simulink model "performMission"  (R2016a)
settings: Solver=VariableStepAuto  StartTime=0.0  StopTime=400  FixedStep=0.001  RelTol=1e-3
InitFcn:
  | workspaceVariablesPerformMission
values from neighbouring files (symbols this model uses):
  ac_id = 127    [goToMission_enu.m]    (also in messageListener.m = 126; workspaceVariablesPerformMissionBackup.m = 202)
  destinations1 = [depot(1,:) ... (first row only)    [workspaceVariablesPerformMission.m]    (also in workspaceVariablesPerformMissionBackup.m = [depot1)
  destinations2 = [depot(2,:) ... (first row only)    [workspaceVariablesPerformMission.m]    (also in workspaceVariablesPerformMissionBackup.m = [depot2)
  pprz_id = 153    [workspaceVariablesPerformMissionBackup.m]
  Q = 3    [workspaceVariablesPerformMission.m]    (also in workspaceVariablesPerformMissionBackup.m)
  wp_ids = [4 5 6 7]    [workspaceVariablesPerformMission.m]    (also in workspaceVariablesPerformMissionBackup.m)
libraries: dspnetwork x4, realtime_pacer_lib x2
settings Model: Creator=pulkit  LastModifiedBy=Kuldeep

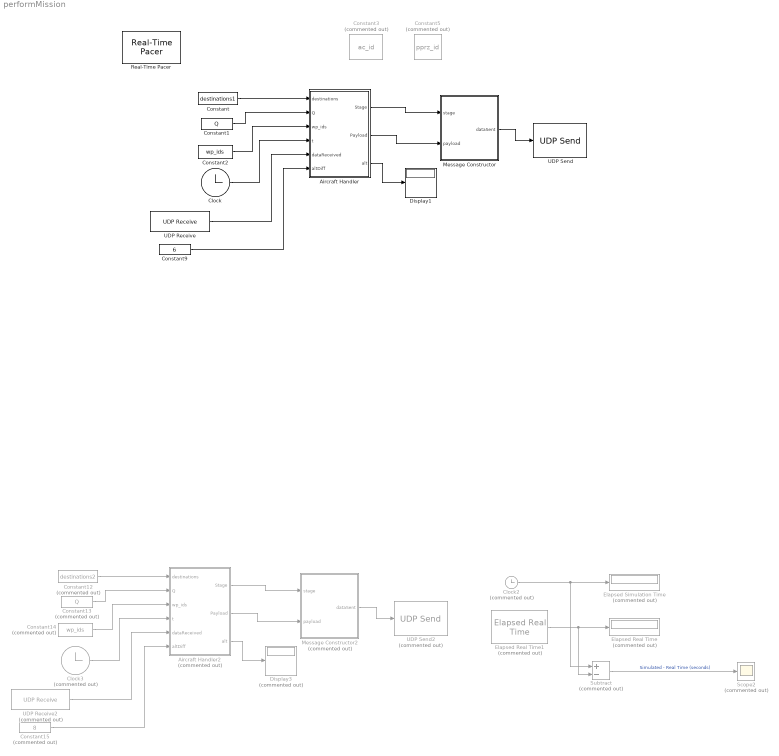
== system performMission ==
  Aircraft Handler : MATLAB Function  TreatAsAtomicUnit=on
  Aircraft Handler2 : MATLAB Function  Commented=on  TreatAsAtomicUnit=on
  Clock : Clock
  Clock2 : Clock  Commented=on
  Clock3 : Clock  Commented=on
  Constant : Constant  Value=destinations1  VectorParams1D=off
  Constant1 : Constant  Value=Q  VectorParams1D=off
  Constant12 : Constant  Commented=on  Value=destinations2  VectorParams1D=off
  Constant13 : Constant  Commented=on  Value=Q  VectorParams1D=off
  Constant14 : Constant  Commented=on  Value=wp_ids  VectorParams1D=off
  Constant15 : Constant  Commented=on  Value=8  VectorParams1D=off
  Constant2 : Constant  Value=wp_ids  VectorParams1D=off
  Constant3 : Constant  Commented=on  Value=ac_id  VectorParams1D=off
  Constant5 : Constant  Commented=on  Value=pprz_id  VectorParams1D=off
  Constant9 : Constant  Value=6  VectorParams1D=off
  Display1 : Display
  Display3 : Display  Commented=on
  Elapsed Real Time : Display  Commented=on
      settings: Decimation=2
  Elapsed Real Time1 : realtime_pacer_lib/Elapsed Real Time  Commented=on
  Elapsed Simulation Time : Display  Commented=on
      settings: Decimation=2
  Message Constructor : MATLAB Function  TreatAsAtomicUnit=on
  Message Constructor2 : MATLAB Function  Commented=on  TreatAsAtomicUnit=on
  Real-Time Pacer : realtime_pacer_lib/Real-Time Pacer  simTimePerRealTime=1
  Scope2 : Scope  Commented=on
  Subtract : Sum  Commented=on  Inputs=+-
  UDP Receive : dspnetwork/UDP Receive  localURL='0.0.0.0'  localPort=4142  remoteURL='0.0.0.0'  remotePort=-1  recvBufferSize=8192  dims=255  signalDatatype=uint8  isVarSize=on  showBlockingTime=on  blockingTime=0.  sampletime=0.005  blockPlatform=HOST
  UDP Receive2 : dspnetwork/UDP Receive  Commented=on  localURL='0.0.0.0'  localPort=4042  remoteURL='0.0.0.0'  remotePort=-1  recvBufferSize=8192  dims=255  signalDatatype=uint8  isVarSize=on  showBlockingTime=on  blockingTime=0.  sampletime=0.005  blockPlatform=HOST
  UDP Send : dspnetwork/UDP Send  remoteURL='255.255.255.255'  remotePort=4143  localURL='0.0.0.0'  localPortSource=Automatically determine  localPort=-1  sampletime=-1  blockPlatform=HOST  separateLengthPort=0
  UDP Send2 : dspnetwork/UDP Send  Commented=on  remoteURL='255.255.255.255'  remotePort=4043  localURL='0.0.0.0'  localPortSource=Automatically determine  localPort=-1  sampletime=-1  blockPlatform=HOST  separateLengthPort=0
  wires:
  Clock/1 -> Aircraft Handler/4(t)
  Constant/1 -> Aircraft Handler/1(destinations)
  Constant1/1 -> Aircraft Handler/2(Q)
  Constant2/1 -> Aircraft Handler/3(wp_ids)
  Aircraft Handler/1(Stage) -> Message Constructor/1(stage)
  Aircraft Handler/2(Payload) -> Message Constructor/2(payload)
  Message Constructor/1(dataSent) -> UDP Send/1
  UDP Receive/1 -> Aircraft Handler/5(dataReceived)
  Clock2/1 -> Subtract/1, Elapsed Simulation Time/1
  Subtract/1 -> Scope2/1  "Simulated - Real Time (seconds)"
  Elapsed Real Time1/1 -> Subtract/2, Elapsed Real Time/1
  Constant9/1 -> Aircraft Handler/6(altDiff)
  Aircraft Handler/3(alt) -> Display1/1
  ? -> ?
  Clock3/1 -> Aircraft Handler2/4(t)
  Constant12/1 -> Aircraft Handler2/1(destinations)
  Constant13/1 -> Aircraft Handler2/2(Q)
  Constant14/1 -> Aircraft Handler2/3(wp_ids)
  Aircraft Handler2/1(Stage) -> Message Constructor2/1(stage)
  Aircraft Handler2/2(Payload) -> Message Constructor2/2(payload)
  Message Constructor2/1(dataSent) -> UDP Send2/1
  UDP Receive2/1 -> Aircraft Handler2/5(dataReceived)
  Constant15/1 -> Aircraft Handler2/6(altDiff)
  Aircraft Handler2/3(alt) -> Display3/1

== matlab function performMission/Aircraft Handler ==
  settings: updateMethod=DISCRETE  sampleTime=0.001
  data: Stage output size=1; destinations input; Payload output size=[1 5]; Q input; wp_ids input; t input; dataReceived input uint8; altDiff input size=[1 1]; alt output size=[1 1]
function [Stage, Payload, alt] = fcn(destinations, Q, wp_ids, t, dataReceived, altDiff)
%#codegen
% This file determines what stage the vehicle is in and forwards the
% appropriate payload. If payload is empty, then no data is sent.

% Following stages are possible:
% % Stage 0 - Initialization (e.g. reading INS_REF)
% % Stage 1 - Event of WP movement i.e. send "MOVE_WP" as payload
% % Stage 2 - Event of instructing vehicle to start following the route i.e.
% send "BLOCK" as payload
% % Stage 3 - Listening when to start the next route. This is decided by
% the user in the flight plan

%% Persistent variables definition
persistent ct_route tStep ct_WP isRouteFinished tol stage stateChange presentRoute alt0 payloadSent

%% Initialize the persistent variables
% % ct_customer - customer number in route for which the WP is being moved

% % ct_route idefies which route number is being currently traversed by the
% vehicle

if isempty(ct_WP)
    ct_WP = 1;
end
if isempty(tStep)
    tStep = 5;
end
if isempty(isRouteFinished)
    isRouteFinished = 1;
end
if isempty(tol)
    tol = 0.001;
end
if isempty(stage)
    stage = 0;
end
if isempty(presentRoute)
    presentRoute = 1;
end
if isempty(ct_route)
    ct_route = 1;
end
if isempty(alt0)
    alt0 = 0;
end
if isempty(payloadSent)
    payloadSent = 0;
end

stateChange = 0;
alt = alt0+altDiff;
ac_id = 126;
block_id = 3; % Start engine block in the flight plan
%% 
% if isRouteFinished && ~isempty(dataReceived) && dataReceived(4)==24
%     val = typecast(dataReceived(5:8), 'single');
%     if abs(val)<tol
%         isRouteFinished = 0;
%     end
% end

% ct_route = floor(t/tStep)+1;

if ct_route <= (size(destinations,1)-1)/Q
    route = [destinations(1,:); destinations((ct_route-1)*Q+2:ct_route*Q+1,:)];
else
    route = destinations(1:Q+1,:);
end

Payload = zeros(1,0);
if stage == 0
    % % Reading the value of reference altitude corresponding to the ground
    % from INS_REF telemetry message
    if ~isempty(dataReceived) && dataReceived(3)==ac_id && dataReceived(4)==154
        alt0 = double(typecast(dataReceived(29:32), 'int32')/1000); % Reading hmsl0
        stage = 40;
        stateChange = 1;
    end
    
elseif stage == 10 % % Update WP for the depot and customers in a route
    % % Move next WP only if the movement of the previous one is confirmed
    % TO DO - change payloadSent to 0 after few seconds (in case message 47
    % is not picked up by the listener)
%     if ~payloadSent
%         coordinates = [route(ct_WP,1:2) alt];
%         wp_id = wp_ids(ct_WP);
%         Payload = [wp_id, ac_id, coordinates];
%         payloadSent = 1;
        
    if ~isempty(dataReceived) && dataReceived(3)==ac_id && dataReceived(4)==47 && dataReceived(5)==wp_ids(ct_WP)
        val = typecast(dataReceived(6:9), 'int32'); % lat
        val1 = typecast(dataReceived(10:13), 'int32'); % lon
        if abs(val-route(ct_WP,1)*10^7)<100 && abs(val1-route(ct_WP,2)*10^7) <100
        %     ct_customer = rem(ct_customer,Q)+1;
            ct_WP = ct_WP + 1;
            if ct_WP > Q+1
                ct_WP = 1;
                stage = 30; 
                stateChange = 1;
            end
        end
        payloadSent = 0;
    end
    coordinates = [route(ct_WP,1:2) alt];
    wp_id = wp_ids(ct_WP);
    Payload = [wp_id, ac_id, coordinates];
    
    
elseif stage == 20 % % Wait for the confirmation from the user to initiate route
    
    
elseif stage == 30 % % Send Start-Engine message and confirm that it happened
    if ~isempty(dataReceived) && dataReceived(3)==ac_id && dataReceived(4)==217
        val = typecast(dataReceived(5:8), 'single');
        if abs(val)<tol % If drone has initiated its route
            stage = 40;
            stateChange = 1;
        else % Send start-engine message
            Payload = [block_id, ac_id];
        end
    end
        
elseif stage == 40 % % Listening till user confirms that drone is ready for next-route
    if ~isempty(dataReceived) && dataReceived(3)==ac_id && dataReceived(4)==217
        val = typecast(dataReceived(5:8), 'single');
        if abs(val-1)<tol
            stage = 10;
            stateChange = 1;
            
            % To change to next route
            ct_route = ct_route+1;
        end
    end
    
end

Stage = stage;
% In case of change in state, the payload is reset to be empty to avoid any
% discrepencies in the datalink message
if stateChange
    Payload = zeros(1,0);
end

== matlab function performMission/Message Constructor ==
  settings: updateMethod=DISCRETE  sampleTime=0.001
  data: stage input; payload input; dataSent output uint8 size=[1 20]
function dataSent = fcn(stage, payload)
%#codegen
% pprz_id - The Paparazzi message ID (Default 153 - Don't change)
% message_id - Message ID of the data to be sent through downlink
% dataL_payload - Length of the payload in Number of bytes (uint8) required
% ac_id - ID of the aircraft to which the message is to be sent
% payload - The actual data to be sent via datalink
% stage - The stage (defined in previous function) at which the present UAV is in
% 
dataSent = uint8(zeros(1,0));
if ~isempty(payload)
    pprz_id = 153;
    dataL_overhead = 4 + 2; % Number of bytes (unint8) required as overhead on actual data
    if stage == 10
        % Construct MOVE_WP message
        message_id = 2;
        dataL_payload = 2 + 4*3;
        dataSent = [uint8(pprz_id) uint8(dataL_overhead+dataL_payload) uint8(0) uint8(message_id) ...
                uint8(payload(1:2)) typecast(int32(payload(3)*10^7),'uint8') typecast(int32(payload(4)*10^7),'uint8') typecast(int32(payload(5)*10^3),'uint8')];
    elseif stage == 30
        % Contruct BLOCK message
        message_id = 5;
        dataL_payload = 2;
        dataSent = [uint8(pprz_id) uint8(dataL_overhead+dataL_payload) uint8(0) uint8(message_id) ...
            uint8(payload(1:2))];
    end

    % Add CHECKSUM if its a useful datalink message
    ck_a = uint8(0);
    ck_b = uint8(0);
    for i=2:dataSent(2)-2
        ck_a = uint8(rem(uint16(ck_a)+uint16(dataSent(i)),uint16(256)));
        ck_b = uint8(rem(uint16(ck_b)+uint16(ck_a),uint16(256)));
    end
    dataSent = typecast([dataSent ck_a ck_b],'uint8');
else
    dataSent = uint8(zeros(1,0));
end

== matlab function performMission/Aircraft Handler2 ==
  settings: updateMethod=DISCRETE  sampleTime=0.001
  data: Stage output size=1; destinations input; Payload output size=[1 5]; Q input; wp_ids input; t input; dataReceived input uint8; altDiff input size=[1 1]; alt output size=[1 1]
function [Stage, Payload, alt] = fcn(destinations, Q, wp_ids, t, dataReceived, altDiff)
%#codegen
% This file determines what stage the vehicle is in and forwards the
% appropriate payload. If payload is empty, then no data is sent.

% Following stages are possible:
% % Stage 0 - Initialization (e.g. reading INS_REF)
% % Stage 1 - Event of WP movement i.e. send "MOVE_WP" as payload
% % Stage 2 - Event of instructing vehicle to start following the route i.e.
% send "BLOCK" as payload
% % Stage 3 - Listening when to start the next route. This is decided by
% the user in the flight plan

%% Persistent variables definition
persistent ct_route tStep ct_WP isRouteFinished tol stage stateChange presentRoute alt0 payloadSent

%% Initialize the persistent variables
% % ct_customer - customer number in route for which the WP is being moved

% % ct_route idefies which route number is being currently traversed by the
% vehicle

if isempty(ct_WP)
    ct_WP = 1;
end
if isempty(tStep)
    tStep = 5;
end
if isempty(isRouteFinished)
    isRouteFinished = 1;
end
if isempty(tol)
    tol = 0.001;
end
if isempty(stage)
    stage = 0;
end
if isempty(presentRoute)
    presentRoute = 1;
end
if isempty(ct_route)
    ct_route = 1;
end
if isempty(alt0)
    alt0 = 0;
end
if isempty(payloadSent)
    payloadSent = 0;
end

stateChange = 0;
alt = alt0+altDiff;
ac_id = 127;
block_id = 3; % Start engine block in the flight plan
%% 
% if isRouteFinished && ~isempty(dataReceived) && dataReceived(4)==24
%     val = typecast(dataReceived(5:8), 'single');
%     if abs(val)<tol
%         isRouteFinished = 0;
%     end
% end

% ct_route = floor(t/tStep)+1;

if ct_route <= (size(destinations,1)-1)/Q
    route = [destinations(1,:); destinations((ct_route-1)*Q+2:ct_route*Q+1,:)];
else
    route = destinations(1:Q+1,:);
end

Payload = zeros(1,0);
if stage == 0
    % % Reading the value of reference altitude corresponding to the ground
    % from INS_REF telemetry message
    if ~isempty(dataReceived) && dataReceived(3)==ac_id && dataReceived(4)==154
        alt0 = double(typecast(dataReceived(29:32), 'int32')/1000); % Reading hmsl0
        stage = 40;
        stateChange = 1;
    end
    
elseif stage == 10 % % Update WP for the depot and customers in a route
    % % Move next WP only if the movement of the previous one is confirmed
    % TO DO - change payloadSent to 0 after few seconds (in case message 47
    % is not picked up by the listener)
%     if ~payloadSent
%         coordinates = [route(ct_WP,1:2) alt];
%         wp_id = wp_ids(ct_WP);
%         Payload = [wp_id, ac_id, coordinates];
%         payloadSent = 1;
        
    if ~isempty(dataReceived) && dataReceived(3)==ac_id && dataReceived(4)==47 && dataReceived(5)==wp_ids(ct_WP)
        val = typecast(dataReceived(6:9), 'int32'); % lat
        val1 = typecast(dataReceived(10:13), 'int32'); % lon
        if abs(val-route(ct_WP,1)*10^7)<100 && abs(val1-route(ct_WP,2)*10^7) <100
        %     ct_customer = rem(ct_customer,Q)+1;
            ct_WP = ct_WP + 1;
            if ct_WP > Q+1
                ct_WP = 1;
                stage = 30; 
                stateChange = 1;
            end
        end
        payloadSent = 0;
    end
    coordinates = [route(ct_WP,1:2) alt];
    wp_id = wp_ids(ct_WP);
    Payload = [wp_id, ac_id, coordinates];
    
    
elseif stage == 20 % % Wait for the confirmation from the user to initiate route
    
    
elseif stage == 30 % % Send Start-Engine message and confirm that it happened
    if ~isempty(dataReceived) && dataReceived(3)==ac_id && dataReceived(4)==217
        val = typecast(dataReceived(5:8), 'single');
        if abs(val)<tol % If drone has initiated its route
            stage = 40;
            stateChange = 1;
        else % Send start-engine message
            Payload = [block_id, ac_id];
        end
    end
        
elseif stage == 40 % % Listening till user confirms that drone is ready for next-route
    if ~isempty(dataReceived) && dataReceived(3)==ac_id && dataReceived(4)==217
        val = typecast(dataReceived(5:8), 'single');
        if abs(val-1)<tol
            stage = 10;
            stateChange = 1;
            
            % To change to next route
            ct_route = ct_route+1;
        end
    end
    
end

Stage = stage;
% In case of change in state, the payload is reset to be empty to avoid any
% discrepencies in the datalink message
if stateChange
    Payload = zeros(1,0);
end

== matlab function performMission/Message Constructor2 ==
  settings: updateMethod=DISCRETE  sampleTime=0.001
  data: stage input; payload input; dataSent output uint8 size=[1 20]
function dataSent = fcn(stage, payload)
%#codegen
% pprz_id - The Paparazzi message ID (Default 153 - Don't change)
% message_id - Message ID of the data to be sent through downlink
% dataL_payload - Length of the payload in Number of bytes (uint8) required
% ac_id - ID of the aircraft to which the message is to be sent
% payload - The actual data to be sent via datalink
% stage - The stage (defined in previous function) at which the present UAV is in
% 
dataSent = uint8(zeros(1,0));
if ~isempty(payload)
    pprz_id = 153;
    dataL_overhead = 4 + 2; % Number of bytes (unint8) required as overhead on actual data
    if stage == 10
        % Construct MOVE_WP message
        message_id = 2;
        dataL_payload = 2 + 4*3;
        dataSent = [uint8(pprz_id) uint8(dataL_overhead+dataL_payload) uint8(0) uint8(message_id) ...
                uint8(payload(1:2)) typecast(int32(payload(3)*10^7),'uint8') typecast(int32(payload(4)*10^7),'uint8') typecast(int32(payload(5)*10^3),'uint8')];
    elseif stage == 30
        % Contruct BLOCK message
        message_id = 5;
        dataL_payload = 2;
        dataSent = [uint8(pprz_id) uint8(dataL_overhead+dataL_payload) uint8(0) uint8(message_id) ...
            uint8(payload(1:2))];
    end

    % Add CHECKSUM if its a useful datalink message
    ck_a = uint8(0);
    ck_b = uint8(0);
    for i=2:dataSent(2)-2
        ck_a = uint8(rem(uint16(ck_a)+uint16(dataSent(i)),uint16(256)));
        ck_b = uint8(rem(uint16(ck_b)+uint16(ck_a),uint16(256)));
    end
    dataSent = typecast([dataSent ck_a ck_b],'uint8');
else
    dataSent = uint8(zeros(1,0));
end
